simulink model "AxialPump"  (R2023b)
settings: Solver=FixedStepAuto  StartTime=0.0  StopTime=t_cycle  FixedStep=1e-8  RelTol=1e-3  EnableMultiTasking=on
InitFcn:
  | %% Outlet
  | % Parameters
  | d_cyl = 8e-3;                                   % Diameter of each piston
  | r_p = 20e-3;                                    % Piston pitch radius
  | A_cyl = 0.25 * pi * d_cyl^2;                    % Area of each piston
  | omega_rpm = 3600;                               % Rotational speed of pump
  | omega = (2*pi/60) * omega_rpm;                  % Angular speed of pump
  | beta = 1.6e9;                                   % Bulk Modulus
  | P1 = 21e6;                                      % Outlet pressure
  | S = 15e-3;                                      % Stroke length
  | Cd = 0.6;                                       % Coefficient of discharge
  | rho = 870;                                      % Density
  | P_T = 101325;                                   % Tank pressure
  | P_P = 21e6;                                     % System pressure
  | c = 10e-6;                                      % Piston-barrel clearance
  | meu = 0.1;                                      % Steel-steel (lubricated) coefficient of friction
  | r2_r1 = 1.6;                                    % Slipper radii ratio
  | r1 = d_cyl/2;
  | do = 0.1e-3;                                    % Slipper orifice opening
  | 
  | % Time parameters
  | theta_cycle = 2 * pi;
  | t_cycle = theta_cycle / omega;
  | theta_t = 2 * asin(d_cyl/(4*r_p));
  | t_t = theta_t/omega;
  | theta_d = theta_cycle/2 - 2 * theta_t;
  | t_d = theta_d/omega;
  | 
  | % Calculated parameters
  | Vdisp = 0.25 * pi * d_cyl^2 * S;
  | Vo = Vdisp;
libraries: SignalEditorBlockLib x2
settings Model: Creator=user  LastModifiedBy=user
settings SolverCC: AutoInsertRateTranBlk=on
settings DataIOCC: SaveOutput=off  SaveTime=off
settings OptimizationCC: DefaultParameterBehavior=Inlined  InlineInvariantSignals=on  EnhancedBackFolding=on  PassReuseOutputArgsAs=Individual arguments  StateBitsets=on  DataBitsets=on  ZeroExternalMemoryAtStartup=off  ZeroInternalMemoryAtStartup=off  NoFixptDivByZeroProtection=on  LifeSpan=1  OptimizeBlockOrder=speed  DifferentSizesBufferReuse=on  EfficientTunableParamExpr=on
settings DebuggingCC: ParameterTunabilityLossMsg=error
settings HardwareCC: ProdBitPerPointer=32  ProdBitPerSizeT=32  ProdBitPerPtrDiffT=32  ProdLargestAtomicFloat=None  ProdIntDivRoundTo=Floor  ProdWordSize=32  ProdHWDeviceType=Generic->Custom
settings SFSimCC: MATLABDynamicMemAlloc=off
settings RTWCC: Description=Embedded Coder  SystemTargetFile=ert.tlc  TLCOptions=-p0  GenCodeOnly=on  TemplateMakefile=ert_default_tmf  GenerateReport=on  RTWVerbose=off  IncludeHyperlinkInReport=on  LaunchReport=on
settings CodeAppCC: ForceParamTrailComments=on  IgnoreCustomStorageClasses=off  OperatorAnnotations=on  SimulinkDataObjDesc=on  SFDataObjDesc=on  CustomSymbolStrGlobalVar=rt$N$M  CustomSymbolStrType=$N$M  CustomSymbolStrFcn=$N$M$F  CustomSymbolStrMacro=$N$M  InsertBlockDesc=on
settings ERTTargetCC: TargetLangStandard=C99 (ISO)  CodeReplacementLibrary=ISO_C  GenerateSampleERTMain=on  IncludeMdlTerminateFcn=off  SuppressErrorStatus=on  SupportAbsoluteTime=off  PurelyIntegerCode=on  SupportNonFinite=off  SupportComplex=off  InlinedParameterPlacement=NonHierarchical  RootIOFormat=Structure reference  ERTCustomFileTemplate=example_file_process.tlc

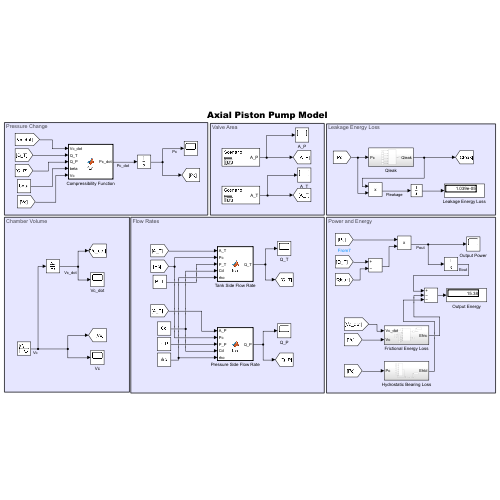
[thumbnail: Simulink's stored preview of the top-level diagram]
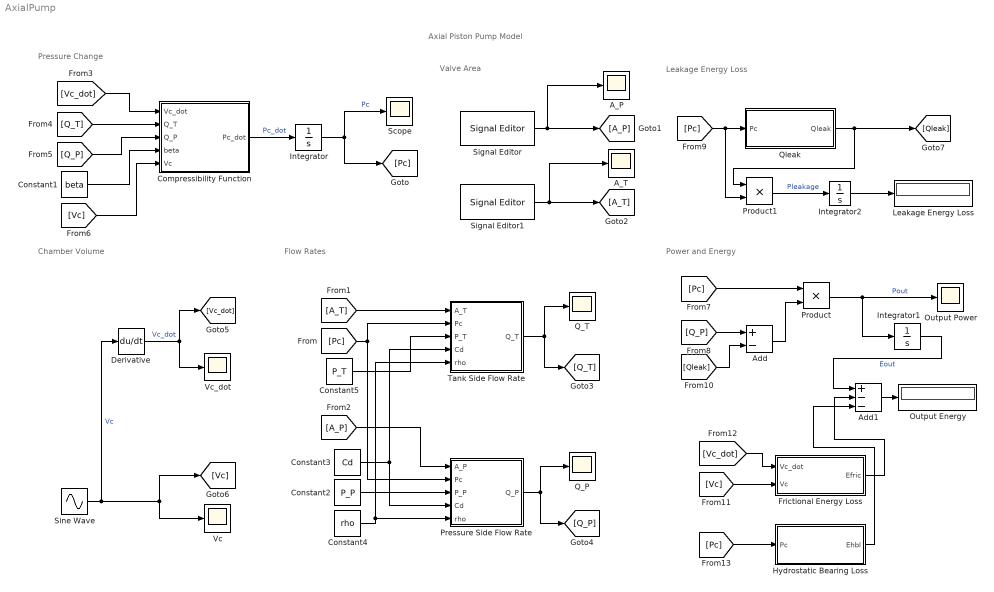
== system AxialPump ==
  note: Power and Energy
  note: Leakage Energy Loss
  note: Pressure Change
  note: Chamber Volume
  note: Valve Area
  note: Flow Rates
  note: Axial Piston Pump Model
      | ​
  A_P : Scope
  A_T : Scope
  Add : Sum  Inputs=+-
  Add1 : Sum  Inputs=+--
  Compressibility Function : MATLAB Function  TreatAsAtomicUnit=on
  Constant1 : Constant  Value=beta
  Constant2 : Constant  Value=P_P
  Constant3 : Constant  Value=Cd
  Constant4 : Constant  Value=rho
  Constant5 : Constant  Value=P_T
  Derivative : Derivative
  Frictional Energy Loss : Subsystem
  Hydrostatic Bearing Loss : Subsystem
  Integrator : Integrator  InitialCondition=P_T
  Integrator1 : Integrator
  Integrator2 : Integrator
  Leakage Energy Loss : Display
  Output Energy : Display
  Output Power : Scope
  Pressure Side Flow Rate : MATLAB Function  TreatAsAtomicUnit=on
  Product : Product
  Product1 : Product
  Q_P : Scope
  Q_T : Scope
  Qleak : Subsystem
  Scope : Scope
  Signal Editor : SignalEditorBlockLib/Signal Editor  FileName=C:\Users\user\OneDrive\Desktop\DR LI\MATLAB\A_T.mat  ActiveScenario=Scenario  ActiveSignal=A_P  IsBus=off  OutputBusObjectStr=Bus: BusObject  SampleTime=0  ZeroCross=off  OutputAfterFinalValue=Setting to zero  Unit=inherit  PreserveSignalName=on  ApplySigPropsToAllScenarios=on  ApplySigPropsToAllSignals=off
  Signal Editor1 : SignalEditorBlockLib/Signal Editor  FileName=C:\Users\user\OneDrive\Desktop\DR LI\MATLAB\A_P.mat  ActiveScenario=Scenario  ActiveSignal=A_T  IsBus=off  OutputBusObjectStr=Bus: BusObject  SampleTime=0  ZeroCross=off  OutputAfterFinalValue=Setting to zero  Unit=inherit  PreserveSignalName=on  ApplySigPropsToAllScenarios=on  ApplySigPropsToAllSignals=off
  Sine Wave : Sin  Amplitude=Vdisp/2  Bias=Vo + (Vdisp/2)  Frequency=omega  Phase=pi/2  SampleTime=0
  Tank Side Flow Rate : MATLAB Function  TreatAsAtomicUnit=on
  Vc : Scope
  Vc_dot : Scope
  wires:
  Signal Editor/1 -> A_P/1, [A_P]
  Sine Wave/1 -> [Vc], Vc/1, Derivative/1  "Vc"
  Derivative/1 -> Vc_dot/1, [Vc_dot]  "Vc_dot"
  Compressibility Function/1(Pc_dot) -> Integrator/1  "Pc_dot"
  Integrator/1 -> [Pc], Scope/1  "Pc"
  Constant1/1 -> Compressibility Function/4(beta)
  Constant2/1 -> Pressure Side Flow Rate/3(P_P)
  Signal Editor1/1 -> [A_T], A_T/1
  Constant3/1 -> Tank Side Flow Rate/4(Cd), Pressure Side Flow Rate/4(Cd)
  Constant4/1 -> Tank Side Flow Rate/5(rho), Pressure Side Flow Rate/5(rho)
  [Pc] -> Pressure Side Flow Rate/2(Pc), Tank Side Flow Rate/2(Pc)
  [A_T] -> Tank Side Flow Rate/1(A_T)
  [A_P] -> Pressure Side Flow Rate/1(A_P)
  Constant5/1 -> Tank Side Flow Rate/3(P_T)
  Tank Side Flow Rate/1(Q_T) -> Q_T/1, [Q_T]
  Pressure Side Flow Rate/1(Q_P) -> Q_P/1, [Q_P]
  [Vc_dot] -> Compressibility Function/1(Vc_dot)
  [Q_T] -> Compressibility Function/2(Q_T)
  [Q_P] -> Compressibility Function/3(Q_P)
  [Vc] -> Compressibility Function/5(Vc)
  [Pc] -> Product/1
  Product/1 -> Integrator1/1, Output Power/1  "Pout"
  Integrator1/1 -> Add1/1  "Eout"
  [Pc] -> Qleak/1(Pc), Product1/2
  Qleak/1(Qleak) -> [Qleak], Product1/1
  Product1/1 -> Integrator2/1  "Pleakage"
  Integrator2/1 -> Leakage Energy Loss/1
  [Q_P] -> Add/1
  Add/1 -> Product/2
  [Qleak] -> Add/2
  Add1/1 -> Output Energy/1
  [Vc_dot] -> Frictional Energy Loss/1(Vc_dot)
  [Vc] -> Frictional Energy Loss/2(Vc)
  Frictional Energy Loss/1(Efric) -> Add1/2
  [Pc] -> Hydrostatic Bearing Loss/1(Pc)
  Hydrostatic Bearing Loss/1(Ehbl) -> Add1/3

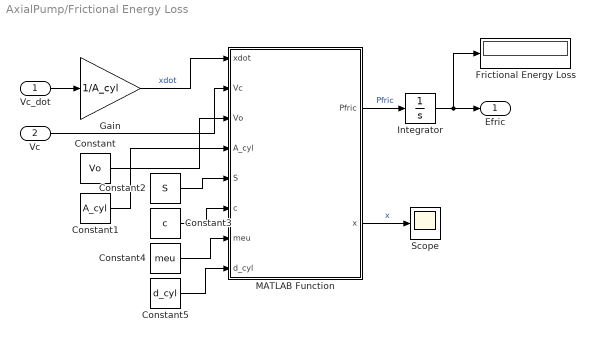
== system AxialPump/Frictional Energy Loss ==
  Vc_dot : Inport
  Vc : Inport  Port=2
  Constant : Constant  Value=Vo
  Constant1 : Constant  Value=A_cyl
  Constant2 : Constant  Value=S
  Constant3 : Constant  Value=c
  Constant4 : Constant  Value=meu
  Constant5 : Constant  Value=d_cyl
  Frictional Energy Loss : Display
  Gain : Gain  Gain=1/A_cyl
  Integrator : Integrator
  MATLAB Function : MATLAB Function  TreatAsAtomicUnit=on
  Scope : Scope
  Efric : Outport
  wires:
  Integrator/1 -> Frictional Energy Loss/1, Efric/1
  Vc_dot/1 -> Gain/1
  Gain/1 -> MATLAB Function/1(xdot)  "xdot"
  MATLAB Function/1(Pfric) -> Integrator/1  "Pfric"
  MATLAB Function/2(x) -> Scope/1  "x"
  Vc/1 -> MATLAB Function/2(Vc)
  Constant/1 -> MATLAB Function/3(Vo)
  Constant1/1 -> MATLAB Function/4(A_cyl)
  Constant2/1 -> MATLAB Function/5(S)
  Constant3/1 -> MATLAB Function/6(c)
  Constant4/1 -> MATLAB Function/7(meu)
  Constant5/1 -> MATLAB Function/8(d_cyl)

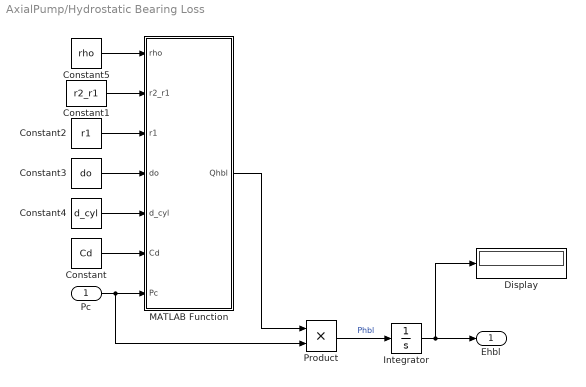
== system AxialPump/Hydrostatic Bearing Loss ==
  Pc : Inport
  Constant : Constant  Value=Cd
  Constant1 : Constant  Value=r2_r1
  Constant2 : Constant  Value=r1
  Constant3 : Constant  Value=do
  Constant4 : Constant  Value=d_cyl
  Constant5 : Constant  Value=rho
  Display : Display
  Integrator : Integrator
  MATLAB Function : MATLAB Function  TreatAsAtomicUnit=on
  Product : Product
  Ehbl : Outport
  wires:
  Constant1/1 -> MATLAB Function/2(r2_r1)
  Constant/1 -> MATLAB Function/6(Cd)
  Constant4/1 -> MATLAB Function/5(d_cyl)
  Constant3/1 -> MATLAB Function/4(do)
  Constant2/1 -> MATLAB Function/3(r1)
  Pc/1 -> Product/2, MATLAB Function/7(Pc)
  MATLAB Function/1(Qhbl) -> Product/1
  Product/1 -> Integrator/1  "Phbl"
  Integrator/1 -> Display/1, Ehbl/1
  Constant5/1 -> MATLAB Function/1(rho)

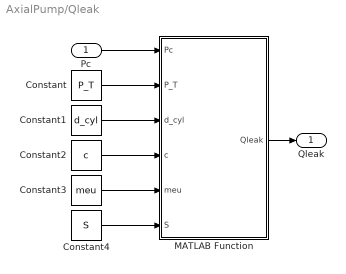
== system AxialPump/Qleak ==
  Pc : Inport
  Constant : Constant  Value=P_T
  Constant1 : Constant  Value=d_cyl
  Constant2 : Constant  Value=c
  Constant3 : Constant  Value=meu
  Constant4 : Constant  Value=S
  MATLAB Function : MATLAB Function  TreatAsAtomicUnit=on
  Qleak : Outport
  wires:
  Pc/1 -> MATLAB Function/1(Pc)
  Constant/1 -> MATLAB Function/2(P_T)
  Constant1/1 -> MATLAB Function/3(d_cyl)
  Constant2/1 -> MATLAB Function/4(c)
  Constant3/1 -> MATLAB Function/5(meu)
  Constant4/1 -> MATLAB Function/6(S)
  MATLAB Function/1(Qleak) -> Qleak/1

== matlab function AxialPump/Tank Side Flow Rate ==
  data: A_T input; Q_T output; Pc input; P_T input; Cd input; rho input
function Q_T = fcn(A_T, Pc, P_T, Cd, rho)

Q_T = Cd*A_T*sqrt((2/rho)*abs(P_T-Pc))*sign(P_T-Pc);

== matlab function AxialPump/Compressibility Function ==
  data: Vc_dot input; Pc_dot output; Q_T input; Q_P input; beta input; Vc input
function Pc_dot = fcn(Vc_dot, Q_T, Q_P, beta, Vc)

Pc_dot = (beta/Vc) * (Q_T - Q_P - Vc_dot);

== matlab function AxialPump/Pressure Side Flow Rate ==
  data: A_P input; Pc input; P_P input; Cd input; rho input; Q_P output
function Q_P = fcn(A_P, Pc, P_P, Cd, rho)

Q_P = Cd*A_P*sqrt((2/rho)*abs(Pc-P_P))*sign(Pc-P_P);

== matlab function AxialPump/Qleak/MATLAB Function ==
  data: Pc input; Qleak output; P_T input; d_cyl input; c input; meu input; S input
function Qleak = fcn(Pc, P_T, d_cyl, c, meu, S)

Qleak = ((0.25*pi*d_cyl^2)*c^3*(Pc-P_T))/(12*meu*S);

== matlab function AxialPump/Frictional Energy Loss/MATLAB Function ==
  data: xdot input; Pfric output; x output; Vc input; Vo input; A_cyl input; S input; c input; meu input; d_cyl input
function [Pfric, x] = fcn(xdot, Vc, Vo, A_cyl, S, c, meu, d_cyl)

x = (Vc - Vo)/A_cyl;
Pfric = (pi*d_cyl*(S-x)*meu*xdot^2)/c;

== matlab function AxialPump/Hydrostatic Bearing Loss/MATLAB Function ==
  data: rho input; r2_r1 input; Qhbl output; r1 input; do input; d_cyl input; Cd input; Pc input
function Qhbl = fcn(rho, r2_r1, r1, do, d_cyl, Cd, Pc)

F_H = 0.25*Pc*pi*d_cyl^2;
Pp = (2*log(r2_r1)*F_H)/(((r2_r1)^2-1)*pi*r1^2);
Qhbl = 0.25*Cd*do^2*sqrt((2/rho)*abs(Pc-Pp))*sign(Pc-Pp);
